simulink model "Model_validate"  (R2020a)
settings: Solver=VariableStepAuto  StartTime=0  StopTime=15  FixedStep=0.001  RelTol=1e-3  AbsTol=1e-6
InitFcn:
  | Lw = 1.6;
  | lf = 1.4;
  | lr = 1.65;
libraries: Solver_SF x1
settings Model: ExtModeTrigMode=oneshot  ExtModeArmWhenConnect=off  Creator=ywata  LastModifiedBy=cksgh
settings SolverCC: AutoScaleAbsTol=off
settings DataIOCC: SaveFormat=Array  ReturnWorkspaceOutputs=off  SignalLoggingName=sigsOut
settings OptimizationCC: BlockReduction=off  BooleanDataType=off  LifeSpan=inf
settings DebuggingCC: SaveWithParameterizedLinksMsg=none  UnderspecifiedInitializationDetection=Classic  MergeDetectMultiDrivingBlocksExec=none  SignalResolutionControl=TryResolveAllWithWarning  MultiTaskDSMMsg=warning  MultiTaskCondExecSysMsg=none  FcnCallInpInsideContextMsg=warning  StateNameClashWarn=warning  SFUnexpectedBacktrackingDiag=warning  SFNoUnconditionalDefaultTransitionDiag=warning  ArithmeticOperatorsInVariantConditions=warning
settings HardwareCC: ProdBitPerPointer=32  ProdBitPerSizeT=32  ProdBitPerPtrDiffT=32  ProdLargestAtomicFloat=None  ProdIntDivRoundTo=Undefined  ProdEndianess=Unspecified  ProdWordSize=32  ProdHWDeviceType=32-bit Generic  TargetUnknown=on
settings ModelReferenceCC: PropagateSignalLabelsOutOfModel=off
settings SFSimCC: SimUseLocalCustomCode=off  CustomCodeUndefinedFunction=UseInterfaceOnly
settings RTWCC: TemplateMakefile=grt_vc.tmf  RTWUseLocalCustomCode=off
settings CodeAppCC: StateflowObjectComments=on
settings GRTTargetCC: TargetFcnLib=ansi_tfl_tmw.mat  TargetLangStandard=C89/C90 (ANSI)  CombineOutputUpdateFcns=off  GRTInterface=on
settings ConfigComp: CovMetricSettings=dw  CovHtmlReporting=on  CovSaveCumulativeToWorkspaceVar=on  CovSaveSingleToWorkspaceVar=on  CovExternalEMLEnable=off

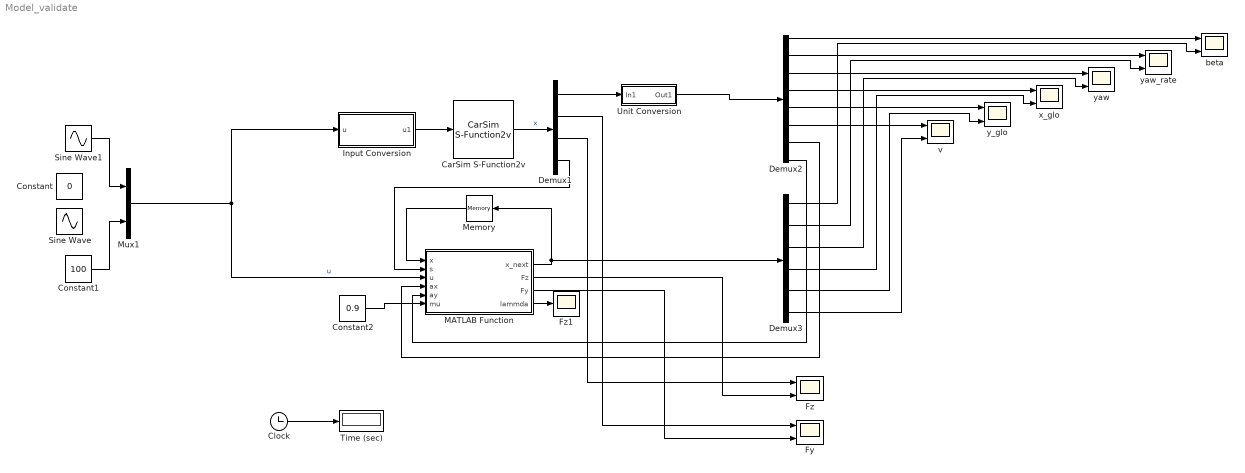
== system Model_validate ==
  CarSim S-Function2v : Solver_SF/CarSim S-Function2v  Priority=1  VehicleCode=i_i  SIMFILE=simfile.sim
      settings: AttributesFormatString=Vehicle Code: %<VehicleCode>
  Clock : Clock
  Constant : Constant  Value=0
  Constant1 : Constant  Value=100
  Constant2 : Constant  Value=0.9
  Demux1 : Demux  Outputs=[8 4 4 4]
  Demux2 : Demux  Outputs=8
  Demux3 : Demux  Outputs=6
  Fy : Scope  NumInputPorts=2
  Fz : Scope  NumInputPorts=2
  Fz1 : Scope
  Input Conversion : Subsystem
  MATLAB Function : MATLAB Function  TreatAsAtomicUnit=on
  Memory : Memory  InitialCondition=[0 0 0 0 -2 16.7]
  Mux1 : Mux  Inputs=2
  Sine Wave : Sin  Amplitude=400  Frequency=2*pi/5  SampleTime=0
  Sine Wave1 : Sin  Amplitude=3*pi/180  Frequency=2*pi/3  SampleTime=0
  Time (sec) : Display
      settings: Format=bank  Decimation=100
  Unit Conversion : Subsystem
  beta : Scope  NumInputPorts=2
  v : Scope  NumInputPorts=2
  x_glo : Scope  NumInputPorts=2
  y_glo : Scope  NumInputPorts=2
  yaw : Scope  NumInputPorts=2
  yaw_rate : Scope  NumInputPorts=2
  wires:
  Clock/1 -> Time (sec)/1
  MATLAB Function/1(x_next) -> Demux3/1, Memory/1
  Mux1/1 -> MATLAB Function/3(u), Input Conversion/1(u)  "u"
  Unit Conversion/1(Out1) -> Demux2/1
  Demux2/1 -> beta/1
  Demux2/6 -> v/1
  Demux2/5 -> y_glo/1
  Demux2/4 -> x_glo/1
  Demux2/3 -> yaw/1
  Demux2/2 -> yaw_rate/1
  Demux3/1 -> beta/2
  Demux3/2 -> yaw_rate/2
  Demux3/3 -> yaw/2
  Demux3/4 -> x_glo/2
  Demux3/5 -> y_glo/2
  Demux3/6 -> v/2
  Sine Wave1/1 -> Mux1/1
  Input Conversion/1(u1) -> CarSim S-Function2v/1
  Memory/1 -> MATLAB Function/1(x)
  CarSim S-Function2v/1 -> Demux1/1  "x"
  Demux1/1 -> Unit Conversion/1(In1)
  Demux2/7 -> MATLAB Function/4(ax)
  Demux2/8 -> MATLAB Function/5(ay)
  Constant2/1 -> MATLAB Function/6(mu)
  MATLAB Function/2(Fz) -> Fz/2
  Demux1/2 -> Fy/1
  Demux1/3 -> Fz/1
  MATLAB Function/3(Fy) -> Fy/2
  Demux1/4 -> MATLAB Function/2(s)
  Constant1/1 -> Mux1/2
  MATLAB Function/4(lammda) -> Fz1/1

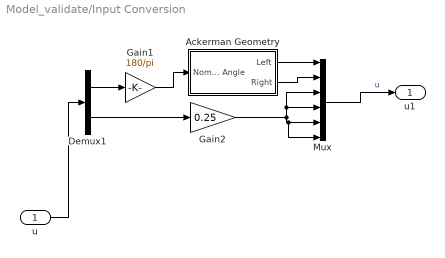
== system Model_validate/Input Conversion ==
  u : Inport
  Ackerman Geometry : Subsystem
  Demux1 : Demux  Outputs=2
  Gain1 : Gain  Gain=180/pi
  Gain2 : Gain  Gain=0.25
  Mux : Mux  Inputs=6
  u1 : Outport
  wires:
  Gain2/1 -> Mux/3, Mux/4, Mux/6, Mux/5
  Mux/1 -> u1/1  "u"
  Ackerman Geometry/1(Left) -> Mux/1
  u/1 -> Demux1/1
  Gain1/1 -> Ackerman Geometry/1(Nominal Angle)
  Demux1/1 -> Gain1/1
  Demux1/2 -> Gain2/1
  Ackerman Geometry/2(Right) -> Mux/2

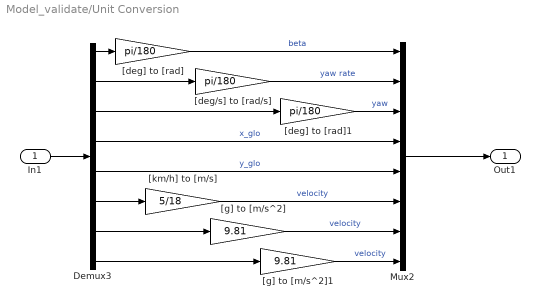
== system Model_validate/Unit Conversion ==
  In1 : Inport
  Demux3 : Demux  Outputs=8
  Mux2 : Mux  Inputs=8
  "[deg/s] to [rad/s]" : Gain  Gain=pi/180
  "[deg] to [rad]" : Gain  Gain=pi/180
  "[deg] to [rad]1" : Gain  Gain=pi/180
  "[g] to [m/s^2]" : Gain  Gain=9.81
  "[g] to [m/s^2]1" : Gain  Gain=9.81
  "[km/h] to [m/s]" : Gain  Gain=5/18
  Out1 : Outport
  wires:
  Demux3/1 -> "[deg] to [rad]"/1
  In1/1 -> Demux3/1
  "[km/h] to [m/s]"/1 -> Mux2/6  "velocity"
  Mux2/1 -> Out1/1
  Demux3/6 -> "[km/h] to [m/s]"/1
  "[deg] to [rad]"/1 -> Mux2/1  "beta"
  Demux3/2 -> "[deg/s] to [rad/s]"/1
  "[deg/s] to [rad/s]"/1 -> Mux2/2  "yaw rate"
  Demux3/3 -> "[deg] to [rad]1"/1
  "[deg] to [rad]1"/1 -> Mux2/3  "yaw"
  Demux3/4 -> Mux2/4  "x_glo"
  Demux3/5 -> Mux2/5  "y_glo"
  Demux3/7 -> "[g] to [m/s^2]"/1
  Demux3/8 -> "[g] to [m/s^2]1"/1
  "[g] to [m/s^2]1"/1 -> Mux2/8  "velocity"
  "[g] to [m/s^2]"/1 -> Mux2/7  "velocity"

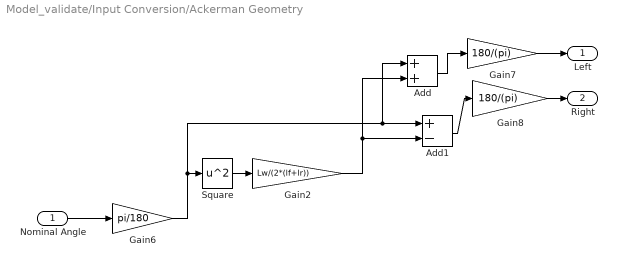
== system Model_validate/Input Conversion/Ackerman Geometry ==
  Nominal Angle : Inport
  Add : Sum
  Add1 : Sum  Inputs=+-
  Gain2 : Gain  Gain=Lw/(2*(lf+lr))
  Gain6 : Gain  Gain=pi/180
  Gain7 : Gain  Gain=180/(pi)
  Gain8 : Gain  Gain=180/(pi)
  Square : Math  Operator=square  SignedPower=on  SaturateOnIntegerOverflow=on
  Left : Outport
  Right : Outport  Port=2
  wires:
  Square/1 -> Gain2/1
  Gain6/1 -> Add/1, Add1/1, Square/1
  Add/1 -> Gain7/1
  Add1/1 -> Gain8/1
  Nominal Angle/1 -> Gain6/1
  Gain7/1 -> Left/1
  Gain8/1 -> Right/1
  Gain2/1 -> Add1/2, Add/2

== matlab function Model_validate/MATLAB Function ==
  data: x input; s input; u input; x_next output; Fz output; Fy output; ax input; ay input; mu input; lammda output
function [x_next, Fz, Fy,lammda] = fcn(x,s,u,ax,ay,mu)
Ts = 0.001;
% [A,B] = myStateJacobian(x,u);
% xdot = A*x + B*u + [0 0 0 0 0 -0.0087*1830*9.81/(1830+4*0.9/0.353^2)]';
[xdot, Fz, Fy,lammda] = nonlinVehicleModel_val(x,s,u,ax,ay,mu);
x_next = x + xdot*Ts;
